simulink model "structured_uncertainty_model"  (R2024b)
settings: Solver=VariableStepAuto  StartTime=0.0  StopTime=10.0  RelTol=1e-3
values from neighbouring files (symbols this model uses):
  Kn = (Ku(1)+Ku(2))/2    [P1.m]
  p1n = (p1u(1)+p1u(2))/2    [P1.m]
  p2n = (p2u(1)+p2u(2))/2    [P1.m]
  Wk = (Ku(2)-Kn)/Kn    [P1.m]
  Wp1 = (p1u(2)-p1n)/p1n    [P1.m]
  Wp2 = (p2u(2)-p2n)/p2n    [P1.m]
settings Model: Creator=lucap  LastModifiedBy=lucap

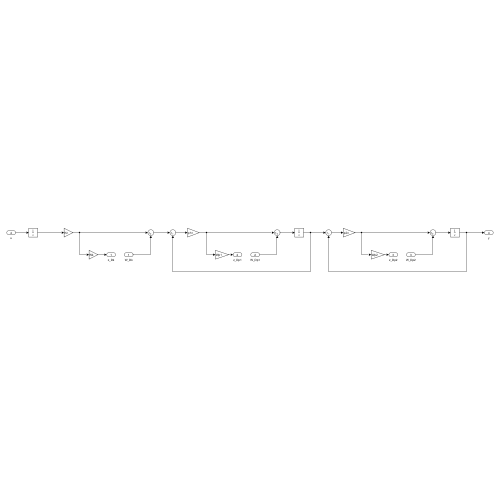
[thumbnail: Simulink's stored preview of the top-level diagram]
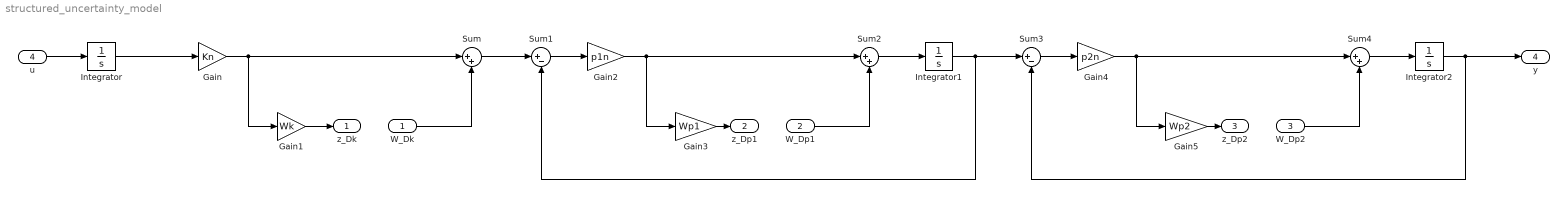
== system structured_uncertainty_model ==
  W_Dk : Inport
  W_Dp1 : Inport  Port=2
  W_Dp2 : Inport  Port=3
  u : Inport  Port=4
  Gain : Gain  Gain=Kn
  Gain1 : Gain  Gain=Wk
  Gain2 : Gain  Gain=p1n
  Gain3 : Gain  Gain=Wp1
  Gain4 : Gain  Gain=p2n
  Gain5 : Gain  Gain=Wp2
  Integrator : Integrator
  Integrator1 : Integrator
  Integrator2 : Integrator
  Sum : Sum  Inputs=|++
  Sum1 : Sum  Inputs=|+-
  Sum2 : Sum  Inputs=|++
  Sum3 : Sum  Inputs=|+-
  Sum4 : Sum  Inputs=|++
  z_Dk : Outport
  z_Dp1 : Outport  Port=2
  z_Dp2 : Outport  Port=3
  y : Outport  Port=4
  wires:
  Integrator/1 -> Gain/1
  Gain1/1 -> z_Dk/1
  Gain/1 -> Gain1/1, Sum/1
  W_Dk/1 -> Sum/2
  Sum/1 -> Sum1/1
  Sum1/1 -> Gain2/1
  Gain3/1 -> z_Dp1/1
  W_Dp1/1 -> Sum2/2
  Gain2/1 -> Gain3/1, Sum2/1
  Sum2/1 -> Integrator1/1
  Integrator1/1 -> Sum3/1, Sum1/2
  Sum3/1 -> Gain4/1
  Sum4/1 -> Integrator2/1
  W_Dp2/1 -> Sum4/2
  Gain4/1 -> Gain5/1, Sum4/1
  Gain5/1 -> z_Dp2/1
  Integrator2/1 -> y/1, Sum3/2
  u/1 -> Integrator/1
